simulink model "BoucingBallCollision"  (R2023a)
settings: Solver=VariableStepAuto  StartTime=0.0  StopTime=60  RelTol=1e-3
libraries: vrlib x2, simulink_extras x1, simulink x1
settings Model: Creator=Personal  LastModifiedBy=Personal

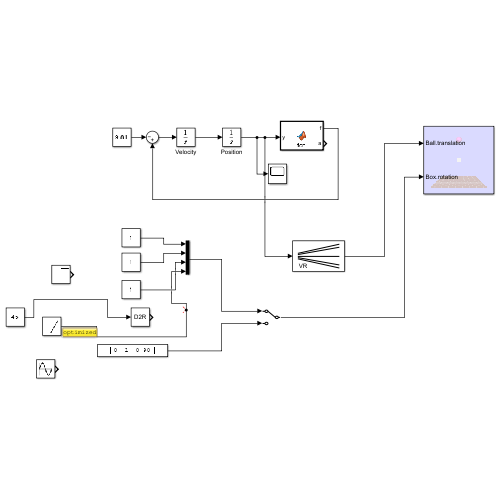
[thumbnail: Simulink's stored preview of the top-level diagram]
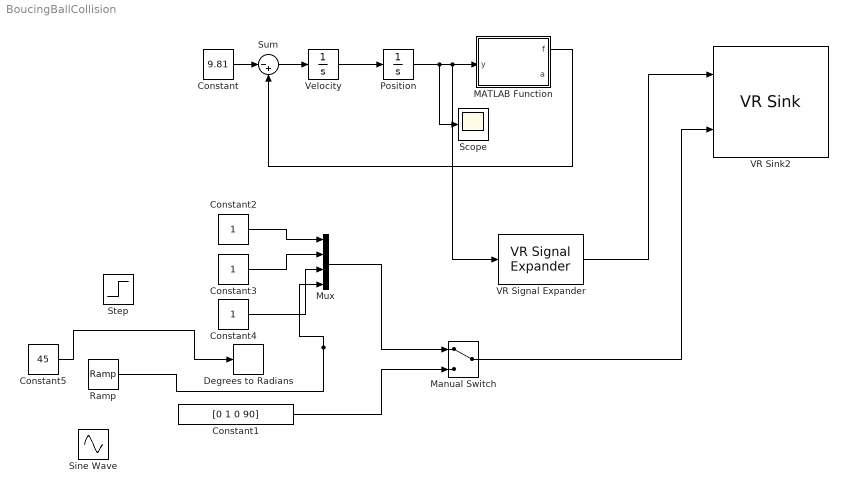
== system BoucingBallCollision ==
  Constant : Constant  Value=9.81
  Constant1 : Constant  Value=[0 1 0 90]
  Constant2 : Constant
  Constant3 : Constant
  Constant4 : Constant
  Constant5 : Constant  Value=45
  Degrees to Radians : simulink_extras/Transformations/Degrees to Radians
  MATLAB Function : MATLAB Function  TreatAsAtomicUnit=on
  Manual Switch : ManualSwitch
  Mux : Mux
  Position : Integrator  InitialCondition=20
  Ramp : simulink/Sources/Ramp  slope=0.1  start=0  InitialOutput=0
  Scope : Scope
  Sine Wave : Sin  Amplitude=2*pi  SampleTime=0
  Step : Step  After=pi/4  SampleTime=0
  Sum : Sum  Inputs=|-+
  VR Signal Expander : vrlib/VR Signal Expander  outwidth=3  outidx=[2]
  VR Sink2 : vrlib/VR Sink  InstantiateOnLoad=on  SampleTime=0.1  ViewEnable=on  RemoteChange=off  RemoteView=off  FieldsWritten=Ball.translation.3.1.1.double#Box.rotation.4.1.1.double  WorldFileName=Ball_Scenario.x3d  AutoView=off  VideoDimensions=[]  AllowVariableSize=off  FigureProperties="{'Position', 'Name', 'Viewpoint', 'CameraBound', 'CameraDirection', 'CameraPosition', 'CameraUpVector', 'ZoomFactor', 'Antialiasing', 'Headlight', 'Lighting', 'NavPanel', 'Sound', 'StatusBar', 'Stereo3D', 'Stereo3DCameraOffset', 'Stereo3DHIT', 'ToolBar', 'Textures', 'Transparency', 'Triad', 'Wireframe', 'NavZones', 'NavMode', 'NavSpeed', 'CaptureFileFormat', 'CaptureFileName', 'Record2DCompressMethod', 'Record2DCompressQuality', 'Record2D', 'Record2DFileName', 'Record2DFPS'; [-1.6790000000000000e+03   3.2800000000000000e+02   1.6800000000000000e+03   8.8300000000000000e+02], '', 'My_viewpoint', 'on', [-7.9849761719484369e-01  -3.2051766078094296e-01  -5.0957824174670441e-01], [2.1624336898543969e+01   7.0380475910549372e+00  -1.5396981818293416e+01], [-2.3866617281366462e-01   9.4566139639712743e-01  -2.2082341659959628e-01], [1.0000000000000000e+00], 'on', 'on', 'on', 'halfbar', 'on', 'on', 'off', [1.0000000149011612e-01], [0.0000000000000000e+00], 'on', 'on', 'on', 'none', 'off', 'off', 'examine', 'normal', 'tif', '%f_anim_%n.tif', 'auto', [7.5000000000000000e+01], 'off', '%f_anim_%n.avi', 'auto'}"
  Velocity : Integrator
  wires:
  Velocity/1 -> Position/1
  Position/1 -> Scope/1, VR Signal Expander/1, MATLAB Function/1(y)
  Sum/1 -> Velocity/1
  Constant/1 -> Sum/1
  MATLAB Function/1(f) -> Sum/2
  VR Signal Expander/1 -> VR Sink2/1
  Manual Switch/1 -> VR Sink2/2
  Constant2/1 -> Mux/1
  Constant3/1 -> Mux/2
  Constant4/1 -> Mux/3
  Constant1/1 -> Manual Switch/2
  Mux/1 -> Manual Switch/1
  Constant5/1 -> Degrees to Radians/1
  Ramp/1 -> Mux/4

== matlab function BoucingBallCollision/MATLAB Function ==
  data: y input; f output; a output
function [f,a] = fcn(y)
if y<1e-4
    y=1e-4;
end
if y<1.5
    f =500*(1.5-y);
    a=sqrt(1.5^3/y);
else
    f=0;
    a=1.5;
end
